simulink model "test"  (R2019b)
settings: Solver=FixedStepAuto  StartTime=0  StopTime=5  FixedStep=1  RelTol=1e-3
settings Model: Creator=yangy  LastModifiedBy=yangy
settings DataIOCC: ExternalInput=aoe_tsinghua_mhi_data  LoadExternalInput=on  SaveFormat=Array  SignalLogging=off
settings OptimizationCC: DefaultParameterBehavior=Inlined  EnhancedBackFolding=on  PassReuseOutputArgsThreshold=0  OptimizeBlockOrder=speed  DifferentSizesBufferReuse=on  OptimizationCustomize=off
settings DebuggingCC: ParameterTunabilityLossMsg=error
settings SFSimCC: MATLABDynamicMemAlloc=off
settings RTWCC: Description=Create Visual C/C++ Solution File for Simulink Coder  TemplateMakefile=RTW.MSVCBuild  GenerateReport=on  LaunchReport=on
settings CodeAppCC: ForceParamTrailComments=on  OperatorAnnotations=on

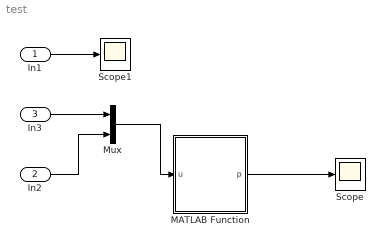
== system test ==
  In1 : Inport  PortDimensions=2
  In2 : Inport  Port=2
  In3 : Inport  Port=3
  MATLAB Function : MATLAB Function  TreatAsAtomicUnit=on
  Mux : Mux  Inputs=2
  Scope : Scope
  Scope1 : Scope
  wires:
  In2/1 -> Mux/2
  Mux/1 -> MATLAB Function/1(u)
  MATLAB Function/1(p) -> Scope/1
  In3/1 -> Mux/1
  In1/1 -> Scope1/1

== matlab function test/MATLAB Function ==
  data: u input; p output
function p = fcn(u)
coder.extrinsic('run_info_recorder','extract_specified_element');
run_info_recorder(extract_specified_element(u,2),[0 1]);
    p = 0;
    if u(1) < 50
        p = 40;
    else
        if u(2) == 50
            p = 600;
        end
        p = p + 60;
    end
end
